simulink model "PRACTICA3"  (R2023a)
settings: Solver=ode15s  StartTime=0.0  StopTime=10  MaxStep=1e-3  RelTol=1e-3
settings Model: Creator=piqui  LastModifiedBy=jaelb
settings DataIOCC: ReturnWorkspaceOutputs=off  TimeSaveName=t
settings DebuggingCC: AlgebraicLoopMsg=none  ArtificialAlgebraicLoopMsg=none  BlockPriorityViolationMsg=error  MinStepSizeMsg=error  MaxConsecutiveZCsMsg=none  ModelReferenceExtraNoncontSigs=none  OperatingPointInterfaceChecksumMismatchMsg=error

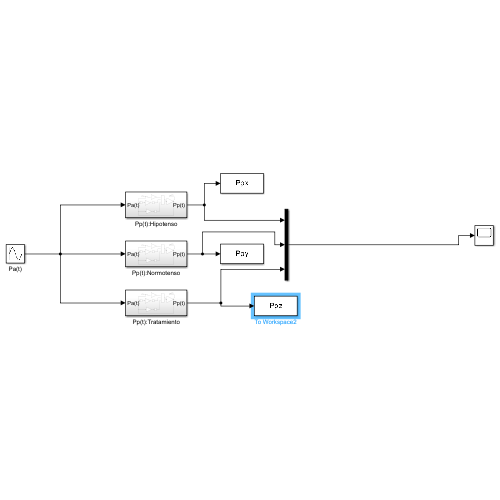
[thumbnail: Simulink's stored preview of the top-level diagram]
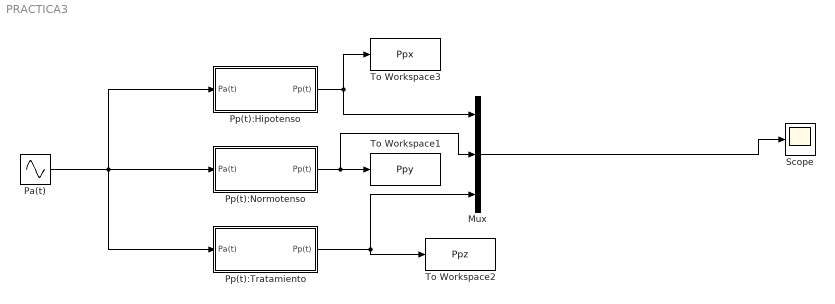
== system PRACTICA3 ==
  Mux : Mux  Inputs=3
  Pa(t) : Sin  Amplitude=2.5  Frequency=2*pi  SampleTime=0
  Pp(t):Hipotenso : Subsystem
  Pp(t):Normotenso : Subsystem
  Pp(t):Tratamiento : Subsystem
  Scope : Scope
  To Workspace1 : ToWorkspace  VariableName=Ppy  SampleTime=-1
  To Workspace2 : ToWorkspace  VariableName=Ppz  SampleTime=-1
  To Workspace3 : ToWorkspace  VariableName=Ppx  SampleTime=-1
  wires:
  Mux/1 -> Scope/1
  Pa(t)/1 -> Pp(t):Hipotenso/1(Pa(t)), Pp(t):Tratamiento/1(Pa(t)), Pp(t):Normotenso/1(Pa(t))
  Pp(t):Hipotenso/1(Pp(t)) -> Mux/1, To Workspace3/1
  Pp(t):Normotenso/1(Pp(t)) -> Mux/2, To Workspace1/1
  Pp(t):Tratamiento/1(Pp(t)) -> To Workspace2/1, Mux/3

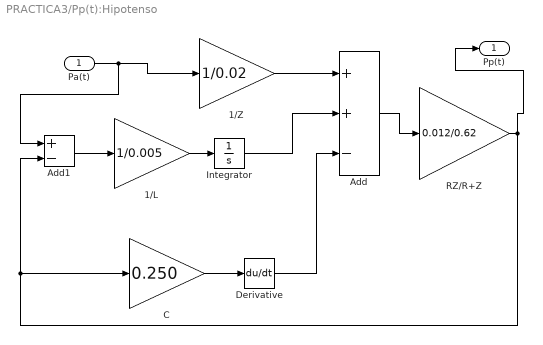
== system PRACTICA3/Pp(t):Hipotenso ==
  Pa(t) : Inport
  1/L : Gain  Gain=1/0.005
  1/Z : Gain  Gain=1/0.02
  Add : Sum  Inputs=++-
  Add1 : Sum  Inputs=+-
  C : Gain  Gain=0.250
  Derivative : Derivative
  Integrator : Integrator
  RZ/R+Z : Gain  Gain=0.012/0.62
  Pp(t) : Outport
  wires:
  RZ/R+Z/1 -> Pp(t)/1, Add1/2, C/1
  Integrator/1 -> Add/2
  1/L/1 -> Integrator/1
  1/Z/1 -> Add/1
  Pa(t)/1 -> Add1/1, 1/Z/1
  C/1 -> Derivative/1
  Derivative/1 -> Add/3
  Add1/1 -> 1/L/1
  Add/1 -> RZ/R+Z/1

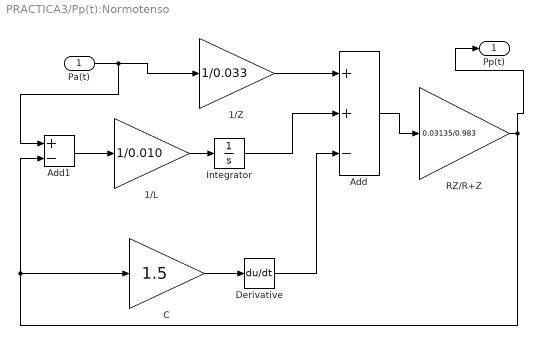
== system PRACTICA3/Pp(t):Normotenso ==
  Pa(t) : Inport
  1/L : Gain  Gain=1/0.010
  1/Z : Gain  Gain=1/0.033
  Add : Sum  Inputs=++-
  Add1 : Sum  Inputs=+-
  C : Gain  Gain=1.5
  Derivative : Derivative
  Integrator : Integrator
  RZ/R+Z : Gain  Gain=0.03135/0.983
  Pp(t) : Outport
  wires:
  Add/1 -> RZ/R+Z/1
  RZ/R+Z/1 -> Pp(t)/1, Add1/2, C/1
  Add1/1 -> 1/L/1
  C/1 -> Derivative/1
  Integrator/1 -> Add/2
  1/L/1 -> Integrator/1
  1/Z/1 -> Add/1
  Pa(t)/1 -> Add1/1, 1/Z/1
  Derivative/1 -> Add/3

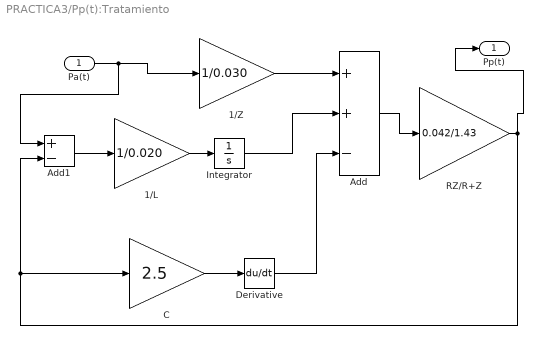
== system PRACTICA3/Pp(t):Tratamiento ==
  Pa(t) : Inport
  1/L : Gain  Gain=1/0.020
  1/Z : Gain  Gain=1/0.030
  Add : Sum  Inputs=++-
  Add1 : Sum  Inputs=+-
  C : Gain  Gain=2.5
  Derivative : Derivative
  Integrator : Integrator
  RZ/R+Z : Gain  Gain=0.042/1.43
  Pp(t) : Outport
  wires:
  Add1/1 -> 1/L/1
  Pa(t)/1 -> Add1/1, 1/Z/1
  1/L/1 -> Integrator/1
  Add/1 -> RZ/R+Z/1
  Derivative/1 -> Add/3
  RZ/R+Z/1 -> Pp(t)/1, Add1/2, C/1
  Integrator/1 -> Add/2
  1/Z/1 -> Add/1
  C/1 -> Derivative/1
